simulink model "work7_5_2"  (R2016a)
settings: Solver=VariableStepAuto  StartTime=0.0  StopTime=20  RelTol=1e-3
settings Model: Creator=AL  LastModifiedBy=AL

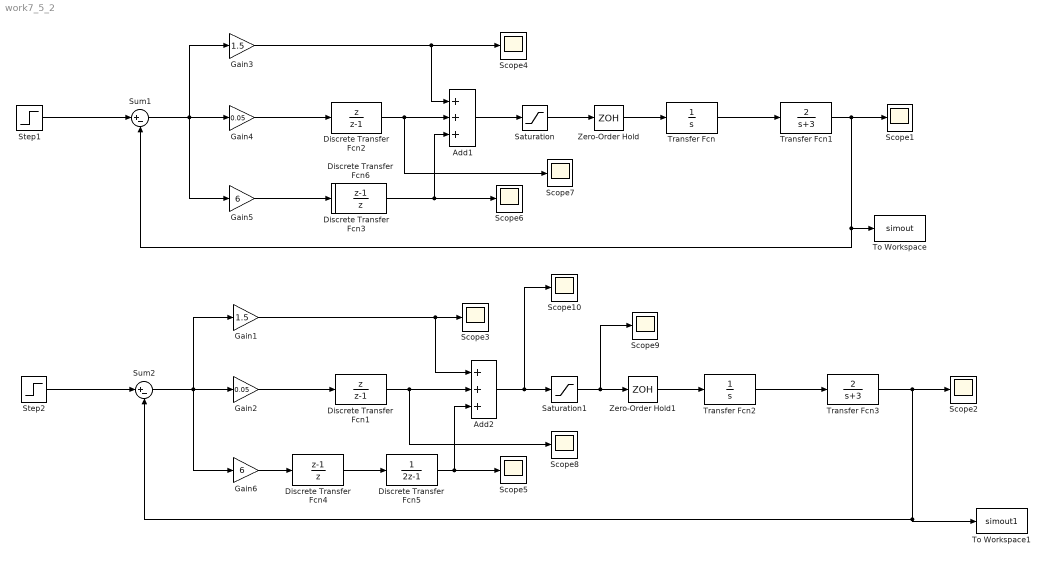
== system work7_5_2 ==
  Add1 : Sum  Inputs=+++
  Add2 : Sum  Inputs=+++
  Discrete Transfer Fcn1 : DiscreteTransferFcn  Numerator=[1 0]  Denominator=[1 -1]  SampleTime=0.1
  Discrete Transfer Fcn2 : DiscreteTransferFcn  Numerator=[1 0]  Denominator=[1 -1]  SampleTime=0.1
  Discrete Transfer Fcn3 : DiscreteTransferFcn  Numerator=[1 -1]  Denominator=[1 0]  SampleTime=0.1
  Discrete Transfer Fcn4 : DiscreteTransferFcn  Numerator=[1 -1]  Denominator=[1 0]  SampleTime=0.1
  Discrete Transfer Fcn5 : DiscreteTransferFcn  Denominator=[2 -1]  SampleTime=0.1
  Discrete Transfer Fcn6 : DiscreteTransferFcn  Numerator=[1 -1]  Denominator=[1 0]  SampleTime=0.1
  Gain1 : Gain  Gain=1.5
  Gain2 : Gain  Gain=0.05
  Gain3 : Gain  Gain=1.5
  Gain4 : Gain  Gain=0.05
  Gain5 : Gain  Gain=6
  Gain6 : Gain  Gain=6
  Saturation : Saturate  UpperLimit=2  LowerLimit=-2
  Saturation1 : Saturate  UpperLimit=2  LowerLimit=-2
  Scope{1..10} (10 alike) : Scope
  Step1 : Step  SampleTime=0
  Step2 : Step  SampleTime=0
  Sum1 : Sum  Inputs=|+-
  Sum2 : Sum  Inputs=|+-
  To Workspace : ToWorkspace  VariableName=simout  SaveFormat=Timeseries  SampleTime=-1
  To Workspace1 : ToWorkspace  VariableName=simout1  SaveFormat=Timeseries  SampleTime=-1
  Transfer Fcn : TransferFcn  Denominator=[1 0]
  Transfer Fcn1 : TransferFcn  Numerator=[2]  Denominator=[1 3]
  Transfer Fcn2 : TransferFcn  Denominator=[1 0]
  Transfer Fcn3 : TransferFcn  Numerator=[2]  Denominator=[1 3]
  Zero-Order Hold : ZeroOrderHold
  Zero-Order Hold1 : ZeroOrderHold
  wires:
  Step1/1 -> Sum1/1
  Sum1/1 -> Gain5/1, Gain4/1, Gain3/1
  Gain3/1 -> Add1/1, Scope4/1
  Gain4/1 -> Discrete Transfer Fcn2/1
  Gain5/1 -> Discrete Transfer Fcn3/1
  Discrete Transfer Fcn2/1 -> Scope7/1, Add1/2
  Discrete Transfer Fcn3/1 -> Add1/3, Scope6/1
  Add1/1 -> Saturation/1
  Saturation/1 -> Zero-Order Hold/1
  Zero-Order Hold/1 -> Transfer Fcn/1
  Transfer Fcn/1 -> Transfer Fcn1/1
  Transfer Fcn1/1 -> Sum1/2, To Workspace/1, Scope1/1
  Step2/1 -> Sum2/1
  Sum2/1 -> Gain6/1, Gain2/1, Gain1/1
  Gain1/1 -> Add2/1, Scope3/1
  Gain2/1 -> Discrete Transfer Fcn1/1
  Gain6/1 -> Discrete Transfer Fcn4/1
  Discrete Transfer Fcn1/1 -> Scope8/1, Add2/2
  Add2/1 -> Scope10/1, Saturation1/1
  Saturation1/1 -> Scope9/1, Zero-Order Hold1/1
  Zero-Order Hold1/1 -> Transfer Fcn2/1
  Transfer Fcn2/1 -> Transfer Fcn3/1
  Transfer Fcn3/1 -> To Workspace1/1, Sum2/2, Scope2/1
  Discrete Transfer Fcn4/1 -> Discrete Transfer Fcn5/1
  Discrete Transfer Fcn5/1 -> Add2/3, Scope5/1
